simulink model "RPI2UdpReceiveTest"  (R2026a)
settings: Solver=FixedStepDiscrete  StopTime=60  FixedStep=rccar.SampleTime
InitFcn:
  | rccarRoot=fileparts(fileparts(fileparts(get_param(bdroot,'FileName')))); addpath(genpath(rccarRoot)); setupRCCarProject; clear rccarRoot;
undefined symbols (not defined in the file): f, rccar
libraries: instrumentlib x1
settings Model: Creator=taegon  LastModifiedBy=taegon

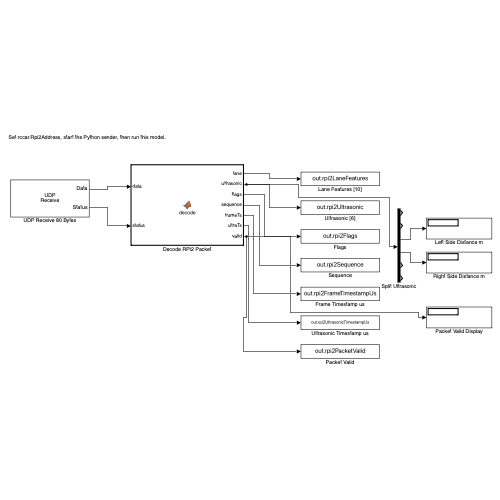
[thumbnail: Simulink's stored preview of the top-level diagram]
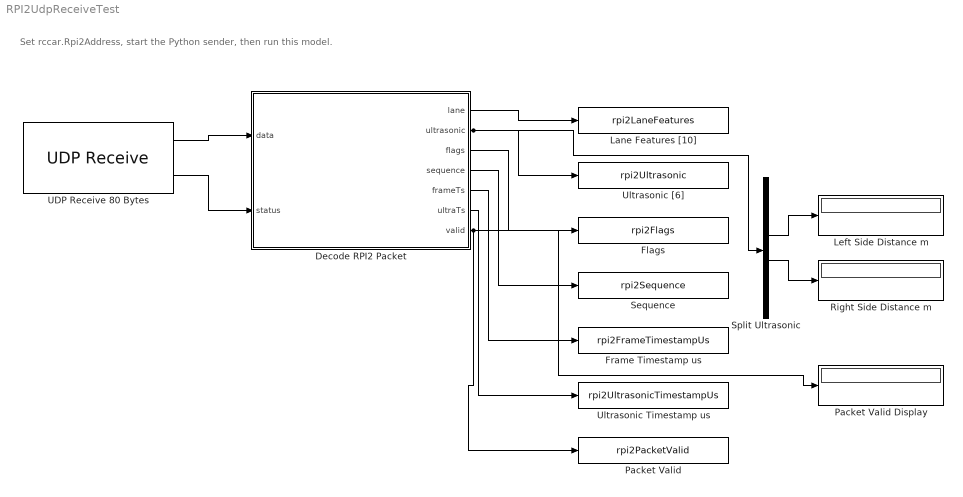
== system RPI2UdpReceiveTest ==
  note: Set rccar.Rpi2Address, start the Python sender, then run this model.
  Decode RPI2 Packet : MATLAB Function  TreatAsAtomicUnit=on
  Flags : ToWorkspace  VariableName=rpi2Flags  SaveFormat=Timeseries  SampleTime=-1
  Frame Timestamp us : ToWorkspace  VariableName=rpi2FrameTimestampUs  SaveFormat=Timeseries  SampleTime=-1
  Lane Features [10] : ToWorkspace  VariableName=rpi2LaneFeatures  SaveFormat=Timeseries  SampleTime=-1
  Left Side Distance m : Display
  Packet Valid : ToWorkspace  VariableName=rpi2PacketValid  SaveFormat=Timeseries  SampleTime=-1
  Packet Valid Display : Display
  Right Side Distance m : Display
  Sequence : ToWorkspace  VariableName=rpi2Sequence  SaveFormat=Timeseries  SampleTime=-1
  Split Ultrasonic : Demux  Outputs=6
  UDP Receive 80 Bytes : instrumentlib/UDP Receive  LocalAddress=0.0.0.0  LocalPort=5005  EnablePortSharing=off  Host=172.30.1.49  Port=5006  GetLatestData=on  DataSize=[80 1]  DataType=uint8  ASCIIFormatting=%f,  Terminator=LF  CustomTerminator=10  ByteOrder=little-endian  EnableBlockingMode=off  Timeout=10  SampleTime=rccar.SampleTime  SimulateUsing=Interpreted execution
  Ultrasonic Timestamp us : ToWorkspace  VariableName=rpi2UltrasonicTimestampUs  SaveFormat=Timeseries  SampleTime=-1
  Ultrasonic [6] : ToWorkspace  VariableName=rpi2Ultrasonic  SaveFormat=Timeseries  SampleTime=-1
  wires:
  UDP Receive 80 Bytes/1 -> Decode RPI2 Packet/1(data)
  UDP Receive 80 Bytes/2 -> Decode RPI2 Packet/2(status)
  Decode RPI2 Packet/1(lane) -> Lane Features [10]/1
  Decode RPI2 Packet/2(ultrasonic) -> Ultrasonic [6]/1, Split Ultrasonic/1
  Decode RPI2 Packet/3(flags) -> Flags/1
  Decode RPI2 Packet/4(sequence) -> Sequence/1
  Decode RPI2 Packet/5(frameTs) -> Frame Timestamp us/1
  Decode RPI2 Packet/6(ultraTs) -> Ultrasonic Timestamp us/1
  Decode RPI2 Packet/7(valid) -> Packet Valid/1, Packet Valid Display/1
  Split Ultrasonic/3 -> Left Side Distance m/1
  Split Ultrasonic/4 -> Right Side Distance m/1

== matlab function RPI2UdpReceiveTest/Decode RPI2 Packet ==
  data: data input; lane output; status input; ultrasonic output; flags output; sequence output; frameTs output; ultraTs output; valid output
function [lane, ultrasonic, flags, sequence, frameTs, ultraTs, valid] = decode(data, status)
%#codegen
persistent heldLane heldSide heldFlags heldSequence heldFrameTs heldUltraTs
if isempty(heldLane)
    heldLane = zeros(10,1,'single'); heldSide = single([NaN;NaN]);
    heldFlags = uint8(0); heldSequence = uint32(0);
    heldFrameTs = uint64(0); heldUltraTs = uint64(0);
end
[newLane, newSide, newFlags, newSequence, newFrameTs, newUltraTs, valid] = rpi2DecodePacket(data, status);
if valid
    heldLane = newLane; heldSide = newSide; heldFlags = newFlags;
    heldSequence = newSequence; heldFrameTs = newFrameTs; heldUltraTs = newUltraTs;
end
lane = heldLane; flags = heldFlags; sequence = heldSequence;
frameTs = heldFrameTs; ultraTs = heldUltraTs;
ultrasonic = single([NaN; NaN; heldSide(1); heldSide(2); NaN; NaN]);
end
